simulink model "jeden_czujnik_arduino"  (R2013a)
settings: Solver=ode45  StartTime=0.0  StopTime=200  RelTol=1e-3
undefined symbols (not defined in the file or in its folder): serial
libraries: instrumentlib x2
settings Model: Creator=Dzientak  LastModifiedBy=Dzientak

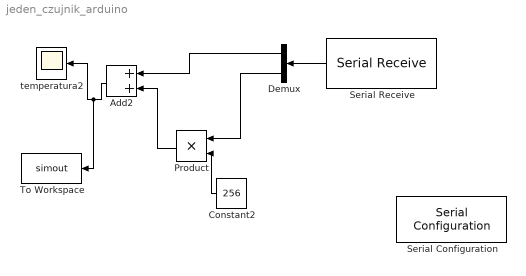
== system jeden_czujnik_arduino ==
  Add2 : Sum
  Constant2 : Constant  Value=256
  Demux : Demux  Outputs=2
  Product : Product
  Serial Configuration : instrumentlib/Serial Configuration  Priority=-200000  ComPortMenu=COM4  ComPort=COM4  ObjConstructor=serial('COM4');  BaudRate=9600  DataBits=8  Parity=none  StopBits=1  FlowControl=none  Timeout=10  ByteOrder=LittleEndian
  Serial Receive : instrumentlib/Serial Receive  ComPortMenu=COM4  ComPort=COM4  ObjConstructor=serial('COM4');  Terminator=<none>  DataSize="[2  1]"  DataType=uint8  EnableBlockingMode=on  ActionDataUnavailable=Output last received value  CustomValue=0  SampleTime=0.01
  To Workspace : ToWorkspace  VariableName=simout  SampleTime=-1  SaveFormat=Timeseries
  temperatura2 : Scope
      settings: ShowLegends=on  TimeRange=200  YMin=35  YMax=120  SaveName=temp1
  wires:
  Serial Receive/1 -> Demux/1
  Constant2/1 -> Product/2
  Demux/2 -> Product/1
  Product/1 -> Add2/2
  Demux/1 -> Add2/1
  Add2/1 -> To Workspace/1, temperatura2/1
